simulink model "cubewithfluid0_pd"  (R2022b)
settings: Solver=VariableStepAuto  StartTime=0.0  StopTime=800  RelTol=1e-3  AbsTol=1e-3
undefined symbols (not defined in the file): tar
settings Model: Creator=Abhijit  LastModifiedBy=abhij
settings SolverCC: AutoScaleAbsTol=off  AlgebraicLoopSolver=TrustRegion  MaxZcPerStep=1
settings DebuggingCC: UnconnectedInputMsg=warning  UnconnectedOutputMsg=warning  UnconnectedLineMsg=warning  SymbolicDimsDataTypeCodeGenerationDiagnostic=none  SFMachineParentedDataDiag=warning
settings ModelReferenceCC: EnableRefExpFcnMdlSchedulingChecks=on
settings SFSimCC: CustomCodeUndefinedFunction=UseInterfaceOnly
settings RTWCC: DLArmComputeVersion=19.05
settings SimscapeCC: SimscapeLogType=all  SimscapeLogSimulationStatistics=on  SimscapeLogDataHistory=10000

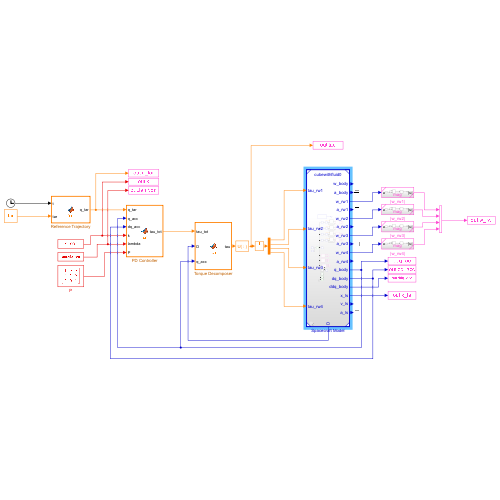
[thumbnail: Simulink's stored preview of the top-level diagram]
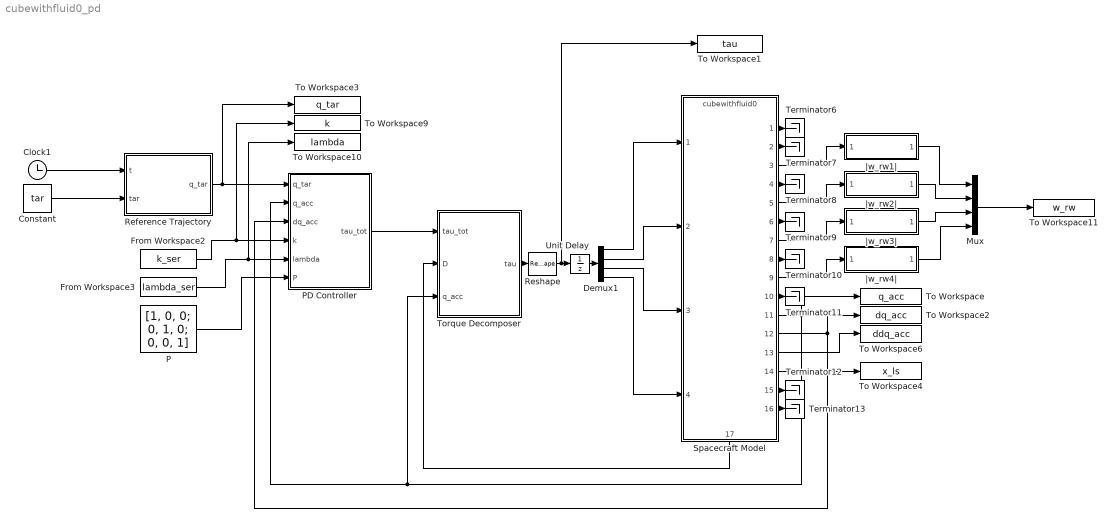
== system cubewithfluid0_pd ==
  Clock1 : Clock
  Constant : Constant  Value=tar
  Demux1 : Demux
  From Workspace2 : FromWorkspace  VariableName=k_ser  Interpolate=off  OutputAfterFinalValue=Holding final value
  From Workspace3 : FromWorkspace  VariableName=lambda_ser
  Mux : Mux
  P : Constant  Value=[1, 0, 0; 0, 1, 0; 0, 0, 1]
  PD Controller : MATLAB Function  TreatAsAtomicUnit=on
  Reference Trajectory : MATLAB Function  TreatAsAtomicUnit=on
  Reshape : Reshape
  Spacecraft Model : ModelReference  ModelNameDialog=cubewithfluid0  SimulationMode=Normal  ModelReferenceVersion=1.23
      settings: PortSchema="{\"entries\":[{\"content\":{\"sides\":[{\"content\":{\"connectorIds\":[\"In1\",\"In2\",\"In3\",\"In4\"]},\"type\":\"ConnectorPlacement.EquallySpacedRectSide\",\"uuid\":\"8e9d2764-0c8c-4b35-a6b5-330d2d8aade7\"},{\"content\":{\"connectorIds\":[\"Out1\",\"Out2\",\"Out3\",\"Out4\",\"Out5\",\"Out6\",\"Out7\",\"Out8\",\"Out9\",\"Out10\",\"Out11\",\"Out12\",\"Out13\",\"Out14\",\"Out15\",\"Out16\"],\"side\":\"RIGHT\"},\"type\":\"ConnectorPlacement.EquallySpacedRectSide\",\"uuid\":\"d11583f7-9081-4803-9c4e-bf58094124c2\"},{\"content\":{\"connectorIds\":[],\"side\":\"TOP\"},\"type\":\"ConnectorPlacement.EquallySpacedRectSide\",\"uuid\":\"f987c09c-5813-428e-a812-016ca0940eea\"},{\"content\":{\"connectorIds\":[\"Out17\"],\"side\":\"BOTTOM\"},\"type\":\"ConnectorPlacement.EquallySpacedRectSide\",\"uuid\":\"56fa612c-373e-46c3-86f2-ebb8be87bff3\"}]},\"type\":\"ConnectorPlacement.EquallySpacedConnector\",\"uuid\":\"9c548295-d181-4ae3-baad-4641f0a6e641\"}],\"packageUris\":[\"http://schema.mathworks.com/mf0/Connector/R2020b\"],\"version\":\"1.0\"}"
  Terminator{6..13} (8 alike) : Terminator
  To Workspace : ToWorkspace  VariableName=q_acc  SaveFormat=Timeseries  SampleTime=-1
  To Workspace1 : ToWorkspace  VariableName=tau  SaveFormat=Timeseries  SampleTime=-1
  To Workspace10 : ToWorkspace  VariableName=lambda  SaveFormat=Timeseries  SampleTime=-1
  To Workspace11 : ToWorkspace  VariableName=w_rw  SaveFormat=Timeseries  SampleTime=-1
  To Workspace2 : ToWorkspace  VariableName=dq_acc  SaveFormat=Timeseries  SampleTime=-1
  To Workspace3 : ToWorkspace  VariableName=q_tar  SaveFormat=Timeseries  SampleTime=-1
  To Workspace4 : ToWorkspace  VariableName=x_ls  SaveFormat=Timeseries  SampleTime=-1
  To Workspace6 : ToWorkspace  VariableName=ddq_acc  SaveFormat=Timeseries  SampleTime=-1
  To Workspace9 : ToWorkspace  VariableName=k  SaveFormat=Timeseries  SampleTime=-1
  Torque Decomposer : MATLAB Function  TreatAsAtomicUnit=on
  Unit Delay : UnitDelay  SampleTime=-1  HasFrameUpgradeWarning=on
  |w_rw1| : Subsystem  ReferencedSubsystem=mag
  |w_rw2| : Subsystem  ReferencedSubsystem=mag
  |w_rw3| : Subsystem  ReferencedSubsystem=mag
  |w_rw4| : Subsystem  ReferencedSubsystem=mag
  wires:
  From Workspace2/1 -> PD Controller/4(k), To Workspace9/1
  Torque Decomposer/1(tau) -> Reshape/1
  From Workspace3/1 -> To Workspace10/1, PD Controller/5(lambda)
  P/1 -> PD Controller/6(P)
  Demux1/3 -> Spacecraft Model/3
  Constant/1 -> Reference Trajectory/2(tar)
  Reference Trajectory/1(q_tar) -> PD Controller/1(q_tar), To Workspace3/1
  Spacecraft Model/11 -> PD Controller/2(q_acc), Torque Decomposer/3(q_acc), To Workspace/1
  Clock1/1 -> Reference Trajectory/1(t)
  Demux1/2 -> Spacecraft Model/2
  Demux1/4 -> Spacecraft Model/4
  Demux1/1 -> Spacecraft Model/1
  Spacecraft Model/12 -> To Workspace2/1, PD Controller/3(dq_acc)
  PD Controller/1(tau_tot) -> Torque Decomposer/1(tau_tot)
  Reshape/1 -> Unit Delay/1, To Workspace1/1
  |w_rw4|/1 -> Mux/4
  |w_rw1|/1 -> Mux/1
  Spacecraft Model/5 -> |w_rw2|/1
  |w_rw2|/1 -> Mux/2
  Spacecraft Model/13 -> To Workspace6/1
  Spacecraft Model/3 -> |w_rw1|/1
  Mux/1 -> To Workspace11/1
  |w_rw3|/1 -> Mux/3
  Spacecraft Model/9 -> |w_rw4|/1
  Spacecraft Model/7 -> |w_rw3|/1
  Spacecraft Model/1 -> Terminator6/1
  Spacecraft Model/2 -> Terminator7/1
  Spacecraft Model/4 -> Terminator8/1
  Spacecraft Model/6 -> Terminator9/1
  Spacecraft Model/8 -> Terminator10/1
  Spacecraft Model/10 -> Terminator11/1
  Unit Delay/1 -> Demux1/1
  Spacecraft Model/14 -> To Workspace4/1
  Spacecraft Model/17 -> Torque Decomposer/2(D)
  Spacecraft Model/15 -> Terminator12/1
  Spacecraft Model/16 -> Terminator13/1

== matlab function cubewithfluid0_pd/PD Controller ==
  data: tau_tot output; q_tar input; q_acc input; dq_acc input; k input; lambda input; P input
function tau_tot = fcn(q_tar, q_acc, dq_acc, k, lambda, P)
    tau_tot = pdcontroller(q_tar, q_acc, dq_acc, k, lambda, P);
end

== matlab function cubewithfluid0_pd/Reference Trajectory ==
  settings: updateMethod=CONTINUOUS
  data: t input; q_tar output; tar input
function q_tar = fcn(t, tar)
     q_tar = refpath(t, tar);
end

== matlab function cubewithfluid0_pd/Torque Decomposer ==
  data: tau_tot input; tau output; D input; q_acc input
function tau = fcn(tau_tot, D, q_acc)
    tau = taudecomp(tau_tot, D, q_acc);
end
